simulink model "Gesamtmodell"  (R2017b)
settings: Solver=ode3  StartTime=0.0  StopTime=inf  FixedStep=dt  RelTol=1e-3  EnableMultiTasking=on
InitFcn:
  | Reglerauslegung
undefined symbols (not defined in the file or in its folder): aMax, aMaxPsi, Blindzeit, Com1, dt, K1, K2, K3, Kx, Ky, none, sigbuilder_block, Tx, Ty, vMax, vMaxPsi
libraries: xpcrtudplib x11, simulink x6, xpcutilitieslib x4, xpcseriallib x1, slrtlib x1
(part 4 of 4)

== matlab function Gesamtmodell/Regelung1/u(x,v)  ==
  data: v1 input; v2 input; v3 input; x1 input; x2 input; x3 input; x4 input; u1 output; u2 output; u3 output; Tx parameter; Ty parameter; Kx parameter; Ky parameter
function [u1, u2, u3]= inputLinearisierung(v1,v2,v3,x1,x2,x3,x4,Tx,Ty,Kx,Ky)


%u1 = (Ty*x1 - Tx*x1 + Ty*v1*cos(x4) + Tx*v2*sin(x4) + Tx*x1*cos(x4)^2 - Ty*x1*cos(x4)^2 - (Tx*x2*sin(2*x4))/2 + (Ty*x2*sin(2*x4))/2 + Tx*Ty*x2*x3)/Ty;
%u2 = -(Ty*x2 - Tx*x2 - Tx*v2*cos(x4) + Ty*v1*sin(x4) + Tx*x2*cos(x4)^2 - Ty*x2*cos(x4)^2 + (Tx*x1*sin(2*x4))/2 - (Ty*x1*sin(2*x4))/2 + Tx*Ty*x1*x3)/Tx;
u1 = (Ty*x1 - Tx*x1 + Tx*x1*cos(x4)^2 - Ty*x1*cos(x4)^2 - (Tx*x2*sin(2*x4))/2 + (Ty*x2*sin(2*x4))/2 + Kx*Ty*v1*cos(x4) + Ky*Tx*v2*sin(x4) + Tx*Ty*x2*x3)/(Kx*Ty);
u2 = -(Ty*x2 - Tx*x2 + Tx*x2*cos(x4)^2 - Ty*x2*cos(x4)^2 + (Tx*x1*sin(2*x4))/2 - (Ty*x1*sin(2*x4))/2 - Ky*Tx*v2*cos(x4) + Kx*Ty*v1*sin(x4) + Tx*Ty*x1*x3)/(Ky*Tx);
u3 = v3;

== matlab function Gesamtmodell/Regelung1/z(x) ==
  data: x1 input; x2 input; x3 input; x4 input; z1 output; z5 output; z2 output; z6 output; x5 input; x6 input; z3 output; z4 output
function [z1,z5,z2,z6,z3,z4]= zustandsTrafo(x1,x2,x3,x4,x5,x6)

z1 = cos(x4) * x1 - sin(x4) * x2;
z2 = sin(x4) * x1 + cos(x4) * x2;
z3 = x3;
z4 = x4;
z5 = x5;
z6 = x6;
